simulink model "LCK_old"  (R2018b)
settings: Solver=FixedStepDiscrete  StartTime=0.0  StopTime=inf  FixedStep=0.005  RelTol=1e-3
PostLoadFcn:
  | if any(exist('dsrtsu_mdlpostloadfcn', 'file') ~= 0), dsrtsu_mdlpostloadfcn('Execute', bdroot); end
values from neighbouring files (symbols this model uses):
  C_DEG2RAD = 0.0175    [LCK_Macro.sldd]
  C_KPH2MPS = 0.2778    [LCK_Macro.sldd]
  C_NEARZERO = 0.0001    [LCK_Macro.sldd]
  C_ONE = 1.0    [LCK_Macro.sldd]
  C_RAD2DEG = 57.2958    [LCK_Macro.sldd]
  C_ZERO = 0.0    [LCK_Macro.sldd]
  k_accel_pedal_pos_per_speed_x : value not decoded    [LCK_LogicPara.sldd]
  k_accel_pedal_pos_per_speed_z : value not decoded    [LCK_LogicPara.sldd]
  k_brake_suprress_hold = 1000.0    [LCK_LogicPara.sldd]
  k_driver_appl_torque_filt = 50.0    [LCK_LogicPara.sldd]
  k_driver_suppression_hold_time = 3000.0    [LCK_LogicPara.sldd]
  k_hands_on_wheel_hold_msec = 500.0    [LCK_LogicPara.sldd]
  k_hands_on_wheel_torque_hi = 0.2    [LCK_LogicPara.sldd]
  k_hands_on_wheel_torque_lo = 0.15    [LCK_LogicPara.sldd]
  k_handsoff_delay_cycles = 50.0    [LCK_LogicPara.sldd]
  k_handsoff_torq_Lo_CR = 0.3    [LCK_LogicPara.sldd]
  k_handson_delay_cycles = 5.0    [LCK_LogicPara.sldd]
  k_HighAccel_suppress_hold = 3000.0    [LCK_LogicPara.sldd]
  k_HLR_suprress_hold = 3000.0    [LCK_LogicPara.sldd]
  k_hs_StrAng_CR_threshold_z : value not decoded    [LCK_LogicPara.sldd]
  k_LC_Exit_Switch = 0.0    [LCK_LogicPara.sldd]
  k_LCG_Configured = 1.0    [LCK_LogicPara.sldd]
  k_LCK_A0_Rdy2Act_UseConst = 0.0    [LCK_LogicPara.sldd]
  k_LCK_A0Fac_ActSta : value not decoded    [LCK_CtrlPara.sldd]
  k_LCK_A0Fac_DrvStm : value not decoded    [LCK_CtrlPara.sldd]
  k_LCK_A0Shift_LftCurv : value not decoded    [LCK_CtrlPara.sldd]
  k_LCK_A0Shift_RgtCurv : value not decoded    [LCK_CtrlPara.sldd]
  k_LCK_A0Shift_StraLan = 0.0    [LCK_CtrlPara.sldd]
  k_LCK_A0ShiftFac_Dy_LftCurv : value not decoded    [LCK_CtrlPara.sldd]
  k_LCK_A0ShiftFac_Dy_RgtCurv : value not decoded    [LCK_CtrlPara.sldd]
  k_LCK_A0ShiftFac_Vspd : value not decoded    [LCK_CtrlPara.sldd]
  k_LCK_accel_inhibit_thold = 35.0    [LCK_LogicPara.sldd]
  k_LCK_Active2Ready_Mask = 255.0    [LCK_LogicPara.sldd]
  k_LCK_CvatRateBks : value not decoded    [LCK_CtrlPara.sldd]
  k_LCK_CvatrBks : value not decoded    [LCK_CtrlPara.sldd]
  k_LCK_DFac_Dy : value not decoded    [LCK_CtrlPara.sldd]
  k_LCK_DFac_Dy_Curv : value not decoded    [LCK_CtrlPara.sldd]
  k_LCK_DFac_HaCurCen : value not decoded    [LCK_CtrlPara.sldd]
  k_LCK_DFac_HaCurSid : value not decoded    [LCK_CtrlPara.sldd]
  k_LCK_DFac_HadCurCen : value not decoded    [LCK_CtrlPara.sldd]
  k_LCK_DFac_HadCurSid : value not decoded    [LCK_CtrlPara.sldd]
  k_LCK_DFac_HadStrCen : value not decoded    [LCK_CtrlPara.sldd]
  k_LCK_DFac_HadStrSid : value not decoded    [LCK_CtrlPara.sldd]
  k_LCK_DFac_HaStrCen : value not decoded    [LCK_CtrlPara.sldd]
  k_LCK_DFac_HaStrSid : value not decoded    [LCK_CtrlPara.sldd]
  k_LCK_DFac_Rad : value not decoded    [LCK_CtrlPara.sldd]
  k_LCK_DFac_SA_CurCen : value not decoded    [LCK_CtrlPara.sldd]
  k_LCK_DFac_SA_CurSid : value not decoded    [LCK_CtrlPara.sldd]
  k_LCK_DFac_SA_StrCen : value not decoded    [LCK_CtrlPara.sldd]
  k_LCK_DFac_SA_StrSid : value not decoded    [LCK_CtrlPara.sldd]
  k_LCK_DFac_SS_CurCen : value not decoded    [LCK_CtrlPara.sldd]
  k_LCK_DFac_SS_CurSid : value not decoded    [LCK_CtrlPara.sldd]
  k_LCK_DFac_SS_StrCen : value not decoded    [LCK_CtrlPara.sldd]
  k_LCK_DFac_SS_StrSid : value not decoded    [LCK_CtrlPara.sldd]
  k_LCK_DFac_Vspd : value not decoded    [LCK_CtrlPara.sldd]
  k_LCK_DlyTm_DrvStim = 0.2    [LCK_CtrlPara.sldd]
  k_LCK_DTermMax = 2.0    [LCK_CtrlPara.sldd]
  k_LCK_DyBks_Curv : value not decoded    [LCK_CtrlPara.sldd]
  k_LCK_Enable_POOnly = 1.0    [LCK_LogicPara.sldd]
  k_LCK_Entry_DistBuffer = 0.1    [LCK_LogicPara.sldd]
  k_LCK_Fac_Vspd2RngThr_FalRec = 0.23    [LCK_CtrlPara.sldd]
  k_LCK_Ffw_CvatSwh = 0.0    [LCK_CtrlPara.sldd]
  k_LCK_Ffw_DyBks : value not decoded    [LCK_CtrlPara.sldd]
  k_LCK_Ffw_TimCon_CmdFlt = 0.0    [LCK_CtrlPara.sldd]
  k_LCK_FfwDeltaFac_Rad_Lft : value not decoded    [LCK_CtrlPara.sldd]
  k_LCK_FfwDeltaFac_Rad_Rgt : value not decoded    [LCK_CtrlPara.sldd]
  k_LCK_FfwDeltaFac_Vspd : value not decoded    [LCK_CtrlPara.sldd]
  k_LCK_FfwFac_CvatRate_Lft : value not decoded    [LCK_CtrlPara.sldd]
  k_LCK_FfwFac_CvatRate_Rgt : value not decoded    [LCK_CtrlPara.sldd]
  k_LCK_FfwFac_Dy : value not decoded    [LCK_CtrlPara.sldd]
  k_LCK_FfwFac_Rad_Lft : value not decoded    [LCK_CtrlPara.sldd]
  k_LCK_FfwFac_Rad_Rgt : value not decoded    [LCK_CtrlPara.sldd]
  k_LCK_FfwFac_Vspd : value not decoded    [LCK_CtrlPara.sldd]
  k_LCK_FfwTorq_Cvat : value not decoded    [LCK_CtrlPara.sldd]
  k_LCK_HAFac_ActSta : value not decoded    [LCK_CtrlPara.sldd]
  k_LCK_HAFac_DrvStm : value not decoded    [LCK_CtrlPara.sldd]
  k_LCK_HaloTime = 2000.0    [LCK_LogicPara.sldd]
  k_LCK_HaloTime_Switch = 0.0    [LCK_LogicPara.sldd]
  k_LCK_HARFac_ActSta : value not decoded    [LCK_CtrlPara.sldd]
  k_LCK_HARFac_DrvStm : value not decoded    [LCK_CtrlPara.sldd]
  k_LCK_Hed_DyBks : value not decoded    [LCK_CtrlPara.sldd]
  k_LCK_HedAngDiffX : value not decoded    [LCK_CtrlPara.sldd]
  k_LCK_HedAngRateDiffX : value not decoded    [LCK_CtrlPara.sldd]
  k_LCK_HndsOnWhel_DlyTm_Idl2Rdy = 0.0    [LCK_LogicPara.sldd]
  k_LCK_host_veh_width = 1.86    [LCK_LogicPara.sldd]
  k_LCK_Idle2Ready_Mask = 239.0    [LCK_LogicPara.sldd]
  k_LCK_Junc_SusTime = 1.0    [LCK_LogicPara.sldd]
  k_LCK_KpKdDecSlopeLmt = 10.0    [LCK_CtrlPara.sldd]
  k_LCK_KpKdIncSlopeLmt = 5.0    [LCK_CtrlPara.sldd]
  k_LCK_Lat_Ctrl_DFac_Lft = 1.0    [LCK_CtrlPara.sldd]
  k_LCK_Lat_Ctrl_DFac_Rgt = 1.05    [LCK_CtrlPara.sldd]
  k_LCK_Lat_Ctrl_Kd = 0.8    [LCK_CtrlPara.sldd]
  k_LCK_Lat_Ctrl_Ki = 0.5    [LCK_CtrlPara.sldd]
  k_LCK_Lat_Ctrl_Kp = 0.7    [LCK_CtrlPara.sldd]
  k_LCK_Lat_Ctrl_Kp_NearGain = 0.7    [LCK_CtrlPara.sldd]
  k_LCK_Lat_Ctrl_PFac_Lft = 1.0    [LCK_CtrlPara.sldd]
  k_LCK_Lat_Ctrl_PFac_Rgt = 1.05    [LCK_CtrlPara.sldd]
  k_LCK_Lat_Ctrl_TimCon_CmdFlt = 5.0    [LCK_CtrlPara.sldd]
  k_LCK_Lat_DFac_Rad : value not decoded    [LCK_CtrlPara.sldd]
  k_LCK_Lat_DFac_SS_Cur : value not decoded    [LCK_CtrlPara.sldd]
  k_LCK_Lat_DFac_SS_Str : value not decoded    [LCK_CtrlPara.sldd]
  k_LCK_Lat_DFac_Vspd : value not decoded    [LCK_CtrlPara.sldd]
  k_LCK_Lat_DyBks : value not decoded    [LCK_CtrlPara.sldd]
  k_LCK_Lat_IFac_Rad : value not decoded    [LCK_CtrlPara.sldd]
  k_LCK_Lat_IFac_Vspd : value not decoded    [LCK_CtrlPara.sldd]
  k_LCK_Lat_ILmtFac_Dy_CurvLan : value not decoded    [LCK_CtrlPara.sldd]
  k_LCK_Lat_ILmtFac_Dy_StraLan : value not decoded    [LCK_CtrlPara.sldd]
  k_LCK_Lat_ILmtFac_Rad : value not decoded    [LCK_CtrlPara.sldd]
  k_LCK_Lat_ILmtFac_Rad_NearGain = 1.0    [LCK_CtrlPara.sldd]
  k_LCK_Lat_ILmtFac_Vspd_CurvLan : value not decoded    [LCK_CtrlPara.sldd]
  k_LCK_Lat_ILmtFac_Vspd_StraLan : value not decoded    [LCK_CtrlPara.sldd]
  k_LCK_Lat_ITermLmt_Dy = 1.0    [LCK_CtrlPara.sldd]
  k_LCK_Lat_KpKdDecSlopeLmt = 10.0    [LCK_CtrlPara.sldd]
  k_LCK_Lat_KpKdIncSlopeLmt = 10.0    [LCK_CtrlPara.sldd]
  k_LCK_Lat_PFac_Dy_InnLftCur : value not decoded    [LCK_CtrlPara.sldd]
  k_LCK_Lat_PFac_Dy_InnRgtCur : value not decoded    [LCK_CtrlPara.sldd]
  k_LCK_Lat_PFac_Dy_OutLftCur : value not decoded    [LCK_CtrlPara.sldd]
  k_LCK_Lat_PFac_Dy_OutRgtCur : value not decoded    [LCK_CtrlPara.sldd]
  k_LCK_Lat_PFac_Dy_Str : value not decoded    [LCK_CtrlPara.sldd]
  k_LCK_Lat_PFac_Rad : value not decoded    [LCK_CtrlPara.sldd]
  ... (+158 more)
undefined symbols (not defined in the file or in its folder): k_LCK_CurvBks, K_LCK_SPA0A1A2_LMRngCmp_y
libraries: LateralControl_fcns_lib x58, simulink x22
(part 12 of 45)

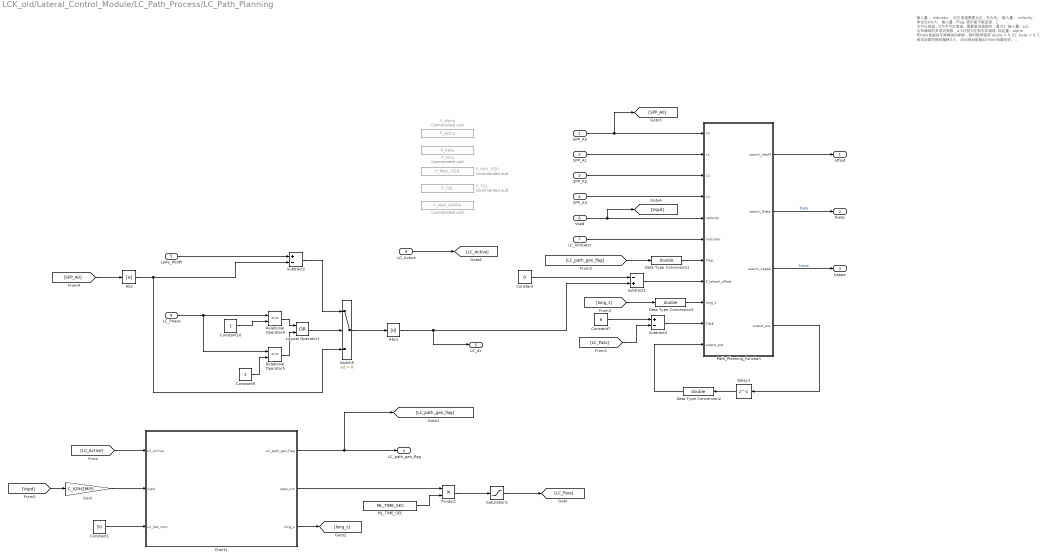
== system LCK_old/Lateral_Control_Module/LC_Path_Process/LC_Path_Planning ==
  note: 输入量： indicator， 向左变道需要为正，右为负。
      | 输入量： velocity, 单位为km/h。
      | 输入量：Flag, 表示能不能变道，1 为可以变道，0为不可以变道。需要激活函数时，置为1.
      | 输入量：a,b 为车辆线的多项式参数，a,b分别为左和右车道线.
      |
      |
      |
      | 标定量：alpha 和beta是曲线平滑模块的参数，暂时推荐使用 alpha = 0.01, beta = 0.7, 测试效果在横向偏移3.5，
      |  纵向规划距离40-80m效果较好。
      | 标定量：P_lateral_offset 是向横向偏移的绝对值，该值取决于路宽和期望的横向偏移的距离。
      | 标定量：P_MAX_ITER 曲线优化的终止条件,这里暂时设置为2000步。
      | 标定量：P_TOL 优化后的曲线与原曲线之间可以接受的最大偏移量，这里推荐使用0.7m
      | 标定量：P_MAX_KAPPA 曲线的优化目标，希望将曲线的曲率下降到某个值以下，这是一个绝对值这里推荐是用0.002,也就是曲率半径500m.
  SPP_A0 : Inport
  SPP_A1 : Inport  Port=2
  SPP_A2 : Inport  Port=3
  SPP_A3 : Inport  Port=4
  Lane_Width : Inport  Port=5
  Vspd : Inport  Port=6
  LC_Indicator : Inport  Port=7
  LC_Active : Inport  Port=8
  LC_Phase : Inport  Port=9
  " " : Constant  Commented=on  Value=P_MAX_KAPPA
  Abs : Abs
  Abs1 : Abs
  Chart1 : Stateflow chart  TreatAsAtomicUnit=on
  Constant : Constant  Value=0
  Constant1 : Constant  Value=50
  Constant10 : Constant
  Constant7 : Constant  Value=6
  Constant9 : Constant  Value=3
  Data Type Conversion1 : DataTypeConversion  OutDataTypeStr=double
  Data Type Conversion2 : DataTypeConversion  OutDataTypeStr=double
  Data Type Conversion3 : DataTypeConversion  OutDataTypeStr=double
  Delay1 : Delay  DelayLength=1  InitialCondition=zeros(400,8)
  Gain : Gain  Gain=C_KPH2MPS
  Logical Operator1 : Logic  Operator=OR  AllPortsSameDT=off  OutDataTypeStr=boolean
  ML_TIME_SEC : Constant  Value=ML_TIME_SEC
  P_MAX_ITER : Constant  Commented=on  Value=P_MAX_ITER
  P_TOL : Constant  Commented=on  Value=P_TOL
  P_alpha : Constant  Commented=on  Value=P_alpha
  P_beta : Constant  Commented=on  Value=P_beta
  "Path_Planning_Function " : MATLAB Function  TreatAsAtomicUnit=on
  Product : Product
  Relational Operator5 : RelationalOperator  Operator===  OutDataTypeStr=boolean  RndMeth=Simplest
  Relational Operator6 : RelationalOperator  Operator===  OutDataTypeStr=boolean  RndMeth=Simplest
  Saturation1 : Saturate  UpperLimit=6  LowerLimit=0
  Subtract1 : Sum  Inputs=-+
  Subtract2 : Sum  Inputs=+-
  Subtract3 : Sum  Inputs=+-
  Switch5 : Switch  Criteria=u2 > Threshold
  offset : Outport
  theta : Outport  Port=2
  kappa : Outport  Port=3
  LC_path_gen_flag : Outport  Port=4
  LC_dx : Outport  Port=5
  wires:
  LC_Indicator/1 -> "Path_Planning_Function "/6(indicator)
  LC_Active/1 -> [LC_Active]
  Vspd/1 -> "Path_Planning_Function "/5(velocity), [Vspd]
  "Path_Planning_Function "/1(search_latoff) -> offset/1
  "Path_Planning_Function "/2(search_theta) -> theta/1  "theta"
  "Path_Planning_Function "/3(search_kappa) -> kappa/1  "kappa"
  Subtract1/1 -> "Path_Planning_Function "/8(P_lateral_offset)
  Constant/1 -> Subtract1/1
  Relational Operator5/1 -> Logical Operator1/2
  Relational Operator6/1 -> Logical Operator1/1
  Constant10/1 -> Relational Operator6/2
  Constant9/1 -> Relational Operator5/2
  LC_Phase/1 -> Relational Operator5/1, Relational Operator6/1
  Logical Operator1/1 -> Switch5/2
  Lane_Width/1 -> Subtract2/1
  [SPP_A0] -> Abs/1
  Abs/1 -> Subtract2/2, Switch5/3
  Subtract2/1 -> Switch5/1
  Switch5/1 -> Abs1/1
  Abs1/1 -> LC_dx/1, Subtract1/2
  Constant7/1 -> Subtract3/1
  Subtract3/1 -> "Path_Planning_Function "/10(TIME)
  [LC_Active] -> Chart1/1(LC_Active)
  Chart1/2(pass_cnt) -> Product/1
  ML_TIME_SEC/1 -> Product/2
  Product/1 -> Saturation1/1
  Chart1/1(LC_path_gen_flag) -> LC_path_gen_flag/1, [LC_path_gen_flag]
  [LC_path_gen_flag] -> Data Type Conversion1/1
  Saturation1/1 -> [LC_Pass]
  [Vspd] -> Gain/1
  Chart1/3(long_s) -> [long_s]
  [long_s] -> Data Type Conversion3/1
  "Path_Planning_Function "/4(output_pre) -> Delay1/1
  Delay1/1 -> Data Type Conversion2/1
  Data Type Conversion2/1 -> "Path_Planning_Function "/11("output_pre ")
  Data Type Conversion1/1 -> "Path_Planning_Function "/7(Flag)
  Data Type Conversion3/1 -> "Path_Planning_Function "/9(long_S)
  Constant1/1 -> Chart1/3(LC_iter_num)
  Gain/1 -> Chart1/2(vspd)
  SPP_A0/1 -> "Path_Planning_Function "/1(c0), [SPP_A0]
  [LC_Pass] -> Subtract3/2
  SPP_A1/1 -> "Path_Planning_Function "/2(c1)
  SPP_A2/1 -> "Path_Planning_Function "/3(c2)
  SPP_A3/1 -> "Path_Planning_Function "/4(c3)

== system LCK_old/Lateral_Control_Module/Steer_Path_Process/Calculation_of_SPP_Confidence ==
  Lin01_Prob_Fltd : Inport
  Lin02_Prob_Fltd : Inport  Port=2
  Constant : Constant  Value=k_LCK_SPPConfHigh_ProbThre
  Constant1 : Constant  Value=4
  Constant2 : Constant  Value=k_LCK_SPPConfMedHigh_ProbThre
  Constant3 : Constant  Value=3
  Constant4 : Constant  Value=k_LCK_SPPConfMed_ProbThre
  Constant5 : Constant  Value=2
  Constant6 : Constant
  Constant7 : Constant  Value=k_LCK_SPPConfHigh_ProbThre
  Constant8 : Constant  Value=k_LCK_SPPConfMedHigh_ProbThre
  Constant9 : Constant  Value=k_LCK_SPPConfMed_ProbThre
  Logical Operator : Logic  AllPortsSameDT=off  OutDataTypeStr=boolean
  Logical Operator1 : Logic  AllPortsSameDT=off  OutDataTypeStr=boolean
  Logical Operator2 : Logic  AllPortsSameDT=off  OutDataTypeStr=boolean
  Relational Operator{,1..5} (6 alike) : RelationalOperator  OutDataTypeStr=boolean  RndMeth=Simplest
  Switch : Switch  Criteria=u2 > Threshold
  Switch1 : Switch  Criteria=u2 > Threshold
  Switch2 : Switch  Criteria=u2 > Threshold
  SPP_Conf_Raw : Outport
  wires:
  Constant6/1 -> Switch2/3
  Lin01_Prob_Fltd/1 -> Relational Operator/1, Relational Operator2/1, Relational Operator1/1
  Logical Operator1/1 -> Switch1/2
  Logical Operator2/1 -> Switch2/2
  Constant8/1 -> Relational Operator4/2
  Constant/1 -> Relational Operator/2
  Logical Operator/1 -> Switch/2
  Constant9/1 -> Relational Operator5/2
  Relational Operator5/1 -> Logical Operator2/2
  Constant3/1 -> Switch1/1
  Constant2/1 -> Relational Operator1/2
  Constant1/1 -> Switch/1
  Relational Operator2/1 -> Logical Operator2/1
  Constant4/1 -> Relational Operator2/2
  Lin02_Prob_Fltd/1 -> Relational Operator3/1, Relational Operator5/1, Relational Operator4/1
  Constant7/1 -> Relational Operator3/2
  Constant5/1 -> Switch2/1
  Relational Operator/1 -> Logical Operator/1
  Relational Operator1/1 -> Logical Operator1/1
  Relational Operator3/1 -> Logical Operator/2
  Switch2/1 -> Switch1/3
  Switch1/1 -> Switch/3
  Relational Operator4/1 -> Logical Operator1/2
  Switch/1 -> SPP_Conf_Raw/1
